simulink subsystem "gibbs2quat"  (R2024b)
settings: Solver=VariableStepAuto  StartTime=0.0  StopTime=10.0  RelTol=1e-3
settings Model: Creator=ricca  LastModifiedBy=ricca

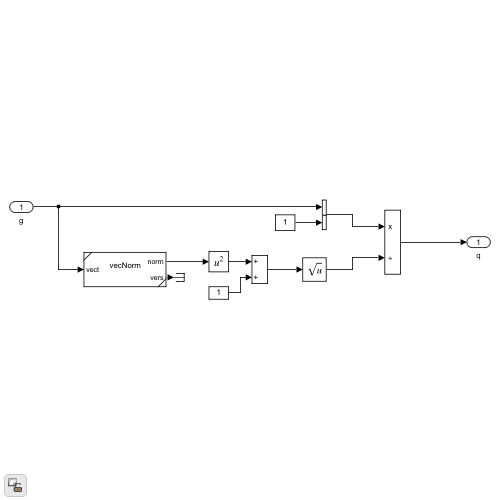
[thumbnail: Simulink's stored preview of the top-level diagram]
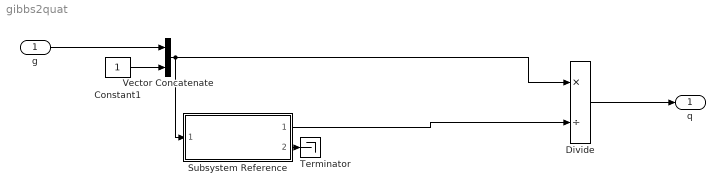
== system gibbs2quat ==
  g : Inport
  Constant1 : Constant
  Divide : Product  Inputs=*/
  Subsystem Reference : Subsystem  ReferencedSubsystem=vecNorm
  Terminator : Terminator
  Vector Concatenate : Concatenate
  q : Outport
  wires:
  g/1 -> Vector Concatenate/1
  Subsystem Reference/2 -> Terminator/1
  Constant1/1 -> Vector Concatenate/2
  Vector Concatenate/1 -> Divide/1, Subsystem Reference/1
  Subsystem Reference/1 -> Divide/2
  Divide/1 -> q/1
